simulink library "NLGCTestSuite"  (R2017b)
settings: Solver=VariableStepAuto  StartTime=0.0  StopTime=10.0  RelTol=1e-3
libraries: simulink x1
settings Model: Creator=hoang  LastModifiedBy=hoang

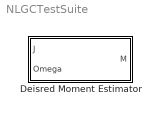
== system NLGCTestSuite ==
  Deisred Moment Estimator : Subsystem  mask{Ts=0}
      mask prompts: Ts "Sampling time (Ts)"

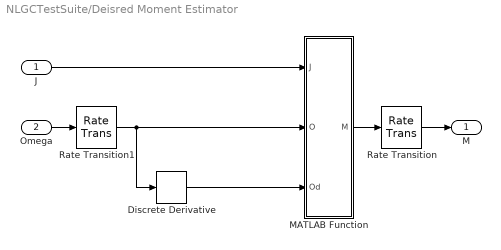
== system NLGCTestSuite/Deisred Moment Estimator ==
  J : Inport
  Omega : Inport  Port=2
  Discrete Derivative : simulink/Discrete/Discrete Derivative  gainval=1.0  ICPrevScaledInput=0.0  OutMin=[]  OutMax=[]  OutDataType=fixdt(1, 16)  OutScaling=2^-10  DoSatur=off
  MATLAB Function : MATLAB Function  TreatAsAtomicUnit=on
  Rate Transition : RateTransition  OutPortSampleTime=Ts
  Rate Transition1 : RateTransition  OutPortSampleTime=Ts
  M : Outport
  wires:
  Omega/1 -> Rate Transition1/1
  J/1 -> MATLAB Function/1(J)
  Discrete Derivative/1 -> MATLAB Function/3(Od)
  MATLAB Function/1(M) -> Rate Transition/1
  Rate Transition/1 -> M/1
  Rate Transition1/1 -> Discrete Derivative/1, MATLAB Function/2(O)

== matlab function NLGCTestSuite/Deisred Moment Estimator/MATLAB Function ==
  data: J input size=[3 3]; M output size=[3 1]; O input size=[3 1]; Od input size=[3 1]
function M = fcn(J,O,Od)
M=dbg_fourth_eqn(J,O,Od)
end
